simulink model "dcIntrocomplete"  (Simulink 8.5)
settings: Solver=ode45  StartTime=0.0  StopTime=Tf  RelTol=1e-3
PreLoadFcn:
  | % Motor Parameters
  | 
  | J=0.01;     %kg*m^2
  | b=0.1;      %N*m/(rad/s)
  | K=0.01;     %V/(rad/s)
  | R=1;        %Ohm
  | L=0.5;      %H
values from neighbouring files (symbols this model uses):
  dist_val = 0.25    [ex7.m]    (also in sim_ex7.m = params.dist_val)
  sat = 50    [ex7.m]    (also in mfunction.m = params.sat; sim_ex7.m = params.sat)
  t0_dist = 10    [ex7.m]    (also in sim_ex7.m = params.t0_vel)
  t0_vel = 5    [ex7.m]    (also in sim_ex7.m = params.t0_vel)
  Ts = 0.01    [ex7.m]    (also in mfunction.m = params.Ts; pid_custom.m; sim_03.m = 0.2; sim_ex7.m = params.Ts)
  variance = 0.0    (= 0)    [ex7.m]    (also in sim_ex7.m = params.variance)
  vel_estat = 3    [ex7.m]    (also in sim_ex7.m = params.vel_estat)
settings Model: Creator=deastman  LastModifiedBy=BPeixoto
settings OptimizationCC: InitFltsAndDblsToZero=on
settings DebuggingCC: SolverPrmCheckMsg=warning  FcnCallInpInsideContextMsg=UseLocalSettings

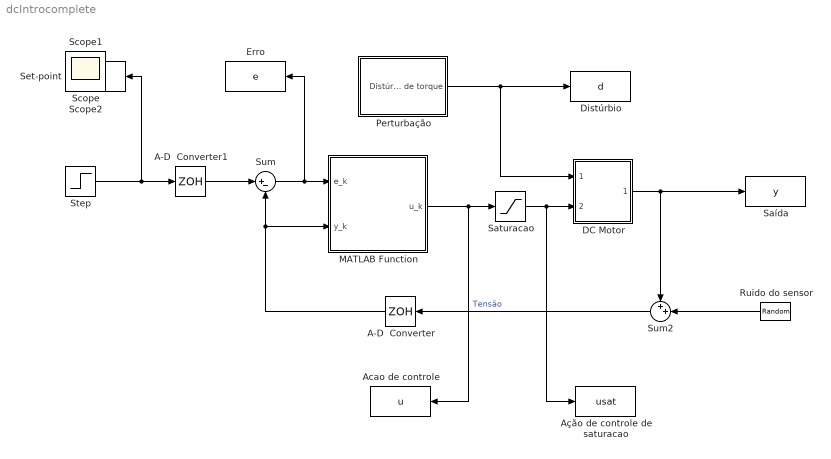
== system dcIntrocomplete ==
  A-D  Converter : ZeroOrderHold  SampleTime=0.02
  A-D  Converter1 : ZeroOrderHold  SampleTime=0.02
  Acao de controle : ToWorkspace  VariableName=u  SaveFormat=Structure With Time  SampleTime=-1
  Ação de controle de saturacao : ToWorkspace  VariableName=usat  SaveFormat=Structure With Time  SampleTime=-1
  DC Motor : Subsystem  mask(DC Motor){b=b, J=J, K=K, R=R, L=L}
      mask prompts: b "Damping:"; J "Inertia:"; K "Back EMF:"; R "Resistance:"; L "Inductance:"
      mask help: An ideal model of a DC Motor
      mask Help: This is <b>more elaborate<b> help.
      mask Display: image(imread('dcmotor.jpg'))
  Distúrbio : ToWorkspace  VariableName=d  SaveFormat=Structure With Time  SampleTime=-1
  Erro : ToWorkspace  VariableName=e  SaveFormat=Structure With Time  SampleTime=-1
  MATLAB Function : MATLAB Function  TreatAsAtomicUnit=on
  Perturbação : Subsystem
  Ruido do sensor : RandomNumber  Variance=variance  SampleTime=Ts
  Saturacao : Saturate  UpperLimit=sat  LowerLimit=-sat
  Saída : ToWorkspace  VariableName=y  SaveFormat=Structure With Time  SampleTime=-1
  Set-point : ToWorkspace  VariableName=w  SaveFormat=Structure With Time  SampleTime=-1
  Step : Step  Time=t0_vel  After=vel_estat  SampleTime=Ts
  Sum : Sum  Inputs=|+-
  Sum2 : Sum  Inputs=++|
  Scope : Scope
      settings: MaxDataPoints=7500
  Scope1 : Scope  NumInputPorts=3
      settings: ShowLegends=on  TimeRange=10  YMin=-3~-60~-0.1  YMax=3~60~0.3  SaveName=ScopeData2  MaxDataPoints=7500
  Scope2 : Scope
      settings: YMin=-50  YMax=50  MaxDataPoints=7500
  wires:
  Sum/1 -> MATLAB Function/1(e_k), Erro/1
  A-D  Converter/1 -> MATLAB Function/2(y_k), Sum/2
  Step/1 -> A-D  Converter1/1, Set-point/1
  A-D  Converter1/1 -> Sum/1
  Ruido do sensor/1 -> Sum2/2
  DC Motor/1(Speed) -> Sum2/1, Saída/1
  Sum2/1 -> A-D  Converter/1
  MATLAB Function/1(u_k) -> Acao de controle/1, Saturacao/1  "Tensão"
  Saturacao/1 -> Ação de controle de saturacao/1, DC Motor/2(Voltage)
  Perturbação/1(Distúrbio de torque) -> Distúrbio/1, DC Motor/1(Torque)

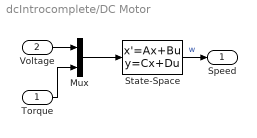
== system dcIntrocomplete/DC Motor ==
  Torque : Inport
  Voltage : Inport  Port=2
  Mux : Mux  Inputs=2
  State-Space : StateSpace  A=[-b/J K/J; -K/L -R/L]  B=[0 -1/J; 1/L 0]  C=[1 0]  D=[0 0]  X0=0
  Speed : Outport
  wires:
  Mux/1 -> State-Space/1
  Voltage/1 -> Mux/1
  State-Space/1 -> Speed/1  "w"
  Torque/1 -> Mux/2

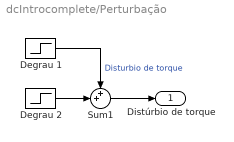
== system dcIntrocomplete/Perturbação ==
  Degrau 1 : Step  Time=t0_dist  After=dist_val  SampleTime=Ts
  Degrau 2 : Step  Time=25  After=-0.25  SampleTime=Ts
  Sum1 : Sum  Inputs=++|
  Distúrbio de torque : Outport
  wires:
  Degrau 1/1 -> Sum1/1  "Disturbio de torque"
  Degrau 2/1 -> Sum1/2
  Sum1/1 -> Distúrbio de torque/1

== matlab function MATLAB Function ==
  data: e_k input double; y_k input double; u_k output double; params parameter double
function u_k = controlador(e_k, y_k, params)

persistent ui_ant;
persistent ud_ant;
persistent u_ant; 
persistent y_ant;

% Atribuicao para primeira iteracao
if isempty(ui_ant) && isempty(ud_ant) && isempty(y_ant)
    ui_ant = 0;
    ud_ant = 0;
    u_ant = 0;
    y_ant = 0;
end

% Parametros do controlador
sat = params.sat;
Ts = params.Ts;
Kp = params.Kp;
Ti = params.Ti;
Td = params.Td;
N = params.N;
a = params.a;

% Erro do integrador
% Estratégia anti-windup
if params.antiwindup
    if (u_ant >= sat) || (u_ant <= -sat)
        ei_k = 0;
    else
        ei_k = e_k;
    end
else
    ei_k = e_k;
end

if (u_ant >= sat)
    e_u = u_ant - sat;
elseif (u_ant <= -sat)
    e_u = u_ant + sat;
else
    e_u = 0;
end

% Saidas e acoes anteriorse
y_k_1 = y_ant;
ui_k_1 = ui_ant;
ud_k_1 = ud_ant;

% Acao proporcional
up_k = Kp*e_k;

% Acao integrativa
ui_k = ui_k_1 + (Kp*Ts/Ti)*ei_k - a*e_u;

% Acao derivativa
ud_k = (Td/(Td + N*Ts))*ud_k_1 - (Kp*N*Td/(Td + N*Ts))*(y_k - y_k_1);

u_k = up_k + ui_k + ud_k;

% Valores salvos para a próxima iteracao
ui_ant = ui_k;
ud_ant = ud_k;
u_ant = u_k;
y_ant = y_k;
